simulink model "schem_1"  (R2024a)
settings: Solver=VariableStepAuto  StartTime=0.0  StopTime=25  MaxStep=1e-4  RelTol=1e-4
undefined symbols (not defined in the file): a0, a1, q0, T, T1, T2
libraries: simulink x1
settings Model: Creator=user  LastModifiedBy=user

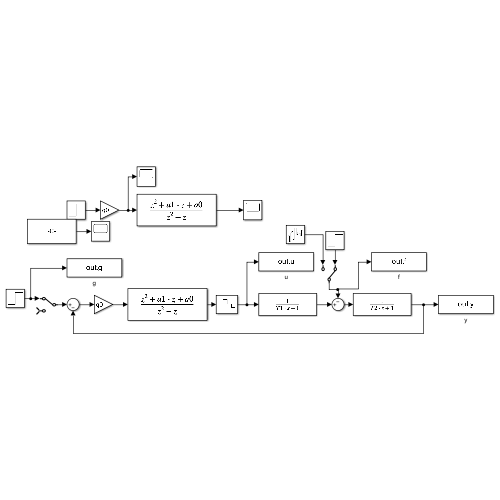
[thumbnail: Simulink's stored preview of the top-level diagram]
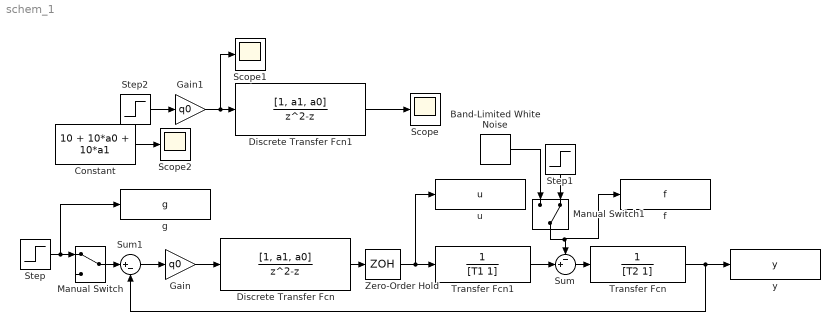
== system schem_1 ==
  Band-Limited White Noise : simulink/Sources/Band-Limited White Noise  Cov=[0.01]  Ts=T  seed=[23341]
  Constant : Constant  Value=10 + 10*a0 + 10*a1
  Discrete Transfer Fcn : DiscreteTransferFcn  Numerator=[1, a1, a0]  Denominator=[1 -1 0]
  Discrete Transfer Fcn1 : DiscreteTransferFcn  Numerator=[1, a1, a0]  Denominator=[1 -1 0]
  Gain : Gain  Gain=q0
  Gain1 : Gain  Gain=q0
  Manual Switch : ManualSwitch
  Manual Switch1 : ManualSwitch  CurrentSetting=0
  Scope : Scope
  Scope1 : Scope
  Scope2 : Scope
  Step : Step  Time=0  SampleTime=0
  Step1 : Step  Time=3  After=2  SampleTime=0
  Step2 : Step  SampleTime=0
  Sum : Sum  Inputs=-+|
  Sum1 : Sum  Inputs=|+-
  Transfer Fcn : TransferFcn  Denominator=[T2 1]
  Transfer Fcn1 : TransferFcn  Denominator=[T1 1]
  Zero-Order Hold : ZeroOrderHold  SampleTime=T
  f : ToWorkspace  VariableName=f  SaveFormat=Timeseries  SampleTime=-1
  g : ToWorkspace  VariableName=g  SaveFormat=Timeseries  SampleTime=-1
  u : ToWorkspace  VariableName=u  SaveFormat=Timeseries  SampleTime=-1
  y : ToWorkspace  VariableName=y  SaveFormat=Timeseries  SampleTime=-1
  wires:
  Step/1 -> g/1, Manual Switch/1
  Manual Switch/1 -> Sum1/1
  Sum1/1 -> Gain/1
  Gain/1 -> Discrete Transfer Fcn/1
  Discrete Transfer Fcn/1 -> Zero-Order Hold/1
  Zero-Order Hold/1 -> u/1, Transfer Fcn1/1
  Transfer Fcn1/1 -> Sum/2
  Sum/1 -> Transfer Fcn/1
  Manual Switch1/1 -> f/1, Sum/1
  Transfer Fcn/1 -> Sum1/2, y/1
  Step1/1 -> Manual Switch1/2
  Band-Limited White Noise/1 -> Manual Switch1/1
  Step2/1 -> Gain1/1
  Discrete Transfer Fcn1/1 -> Scope/1
  Constant/1 -> Scope2/1
  Gain1/1 -> Scope1/1, Discrete Transfer Fcn1/1
